simulink model "Engine_Testrig"  (R2013b)
settings: Solver=ode15s  StartTime=0.0  StopTime=100  RelTol=1e-5  AbsTol=1e-4
undefined symbols (not defined in the file): HEV_Param
libraries: fl_lib x10, nesl_utility x5, sdl_lib x1, simulink x1
Description:
  | Copyright 2015 The MathWorks, Inc.
settings Model: Creator=smiller  LastModifiedBy=smiller
settings DataIOCC: SignalLoggingSaveFormat=ModelDataLogs
settings OptimizationCC: ExpressionDepthLimit=2147483647
settings DebuggingCC: FcnCallInpInsideContextMsg=UseLocalSettings  StateNameClashWarn=warning
settings GRTTargetCC: CombineOutputUpdateFcns=off  GRTInterface=on

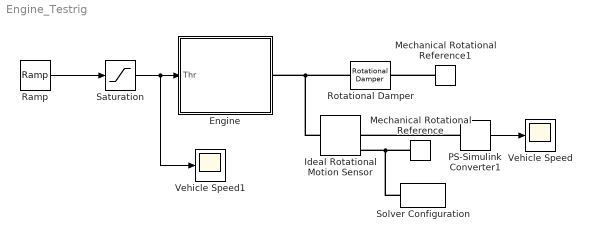
== system Engine_Testrig ==
  Engine : Subsystem
      mask Display:
      | image(imread('HEV_Engine_IMAGE.jpg'));
      | port_label('input',1,'Thr');
      | port_label('RConn',1,'Sh');
  Ideal Rotational Motion Sensor : fl_lib/Mechanical/Mechanical Sensors/Ideal Rotational Motion Sensor  offset=0 rad  w_Log=off  t_Log=off  phi_Log=off  LocalVarNames=|w|t|phi  LocalVarDescs=|w|t|phi  LocalVarLogging=[0 0 0]
  Mechanical Rotational Reference : fl_lib/Mechanical/Rotational Elements/Mechanical Rotational Reference  t_Log=off  LocalVarNames=|t  LocalVarDescs=|t  LocalVarLogging=0
  Mechanical Rotational Reference1 : fl_lib/Mechanical/Rotational Elements/Mechanical Rotational Reference  t_Log=off  LocalVarNames=|t  LocalVarDescs=|t  LocalVarLogging=0
  PS-Simulink Converter1 : nesl_utility/PS-Simulink Converter  PhysicalDomain=network_engine_domain  SubClassName=ps_output  LeftPortType=input  RightPortType=output  PseudoPeriodic=off  Frequencies=[]  Unit=rpm  AffineConversion=off
  Ramp : simulink/Sources/Ramp  slope=0.1  start=0.1  X0=0
  Rotational Damper : fl_lib/Mechanical/Rotational Elements/Rotational Damper  D=HEV_Param.ICE.Friction*0.001 N*m/(rad/s)  t_Log=off  w_Log=off  LocalVarNames=|t|w  LocalVarDescs=|t|w  LocalVarLogging=[0 0]
  Saturation : Saturate  UpperLimit=1  LowerLimit=-1
  Solver Configuration : nesl_utility/Solver Configuration  PhysicalDomain=network_engine_domain  SubClassName=solver  LeftPortType=input  RightPortType=generic  Accelerate=off  Tones=[]  Harmonics=[]  SimulateNoise=off  Profile=off  UseLocalSampling=off  EnableSwitchedLinearOptims=on  FrequencyDomain=off  UseCCode=off  RelTol=0.001  AbsTol=1e-06  MinStep=1e-09  ToWorkspace=off  DoDC=off  ResidualTolerance=1e-9  UseLocalSolver=off  LocalSolverChoice=NE_BACKWARD_EULER_ADVANCER  LocalSolverSampleTime=0.005  DoFixedCost=off  MaxNonlinIter=3  MaxModeIter=2  LinearAlgebra=Sparse  DelaysMemoryBudget=1024
  Vehicle Speed : Scope
      settings: YMin=0  YMax=120  Decimation=decimation
  Vehicle Speed1 : Scope
      settings: YMin=0  YMax=120  Decimation=decimation
  wires:
  Ramp/1 -> Saturation/1
  Saturation/1 -> Engine/1(Thr), Vehicle Speed1/1
  PS-Simulink Converter1/1 -> Vehicle Speed/1
  connections:
  Ideal Rotational Motion Sensor/LConn1 -- Engine/RConn1 -- Rotational Damper/LConn1
  Mechanical Rotational Reference1/LConn1 -- Rotational Damper/RConn1
  PS-Simulink Converter1/LConn1 -- Ideal Rotational Motion Sensor/RConn2
  Mechanical Rotational Reference/LConn1 -- Ideal Rotational Motion Sensor/RConn1 -- Solver Configuration/RConn1

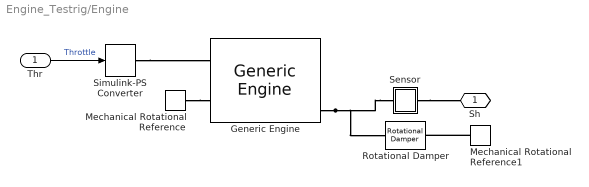
== system Engine_Testrig/Engine ==
  Thr : Inport
  Generic Engine : sdl_lib/Engines/Generic Engine  model_parameterization=1  engine_type=1  P_max=HEV_Param.ICE.Max_Power W  w_P_max=HEV_Param.ICE.Speed_At_Max_Power rpm  w_max=HEV_Param.ICE.Max_Speed rpm  w_min=500 rpm  w_tab=[ 500 1000 2e+3 3e+3 4e+3 5e+3 6e+3 7e+3 ] rpm  trq_tab=[ 380 380 380 380 350 280 200 80 ] N*m  pwr_tab=[ 2e+4 4e+4 7.8e+4 1.2e+5 1.45e+5 1.48e+5 1.25e+5 6e+4 ] W  interp_method=1  model_inertia=1  inertia=HEV_Param.ICE.Shaft_Inertia kg*m^2  initial_velocity=800 rpm  model_time_constant=0  time_constant=0.2 s  T0=0  w_thr=100 rpm  idle_speed=0  idle_speed_reference=1000 rpm  tau_controller=1 s  idle_w_thr=1 rpm  fc_model=1  fc_per_rev=25 mg/rev  displaced_volume=400 cm^3  rev_per_cycle=2  fc_w_tab=[ 1000 2e+3 3e+3 4e+3 5e+3 6e+3 ] rpm  fc_trq_tab=[ 0 80 160 200 240 320 360 400 ] N*m  fc_tab=[ 0.5 0.9 1.4 1.6 1.9 2.7 3.4 4.4; 1 1.7 2.7 3.1 3.6 5 6 7.4; 1.4 2.7 4 4.8 5.6 7.5 8.5 10.5; 2 3.6 5.8 6.7 8 10.4 11.7 13.3; 2.5 4.8 7.9 9.4 10.8 14 16.2 18.6; 3.1 6 10.3 11.9 13.8 18.4 22 26.5 ] g/s  bmep_tab=[ 0 250 500 625 750 1000 1.15e+3 1.25e+3 ] kPa  bsfc_tab=[ 410 380 300 280 270 290 320 380; 410 370 290 270 260 270 285 320; 415 380 290 275 265 270 270 300; 420 390 310 290 285 280 280 285; 430 410 340 320 310 300 310 320; 450 430 370 340 330 330 350 380 ] g/hr/kW  fc_interp_method=1  LocalVarLogging=[]
  Mechanical Rotational Reference : fl_lib/Mechanical/Rotational Elements/Mechanical Rotational Reference  t_Log=off  LocalVarNames=|t  LocalVarDescs=|t  LocalVarLogging=0
  Mechanical Rotational Reference1 : fl_lib/Mechanical/Rotational Elements/Mechanical Rotational Reference  t_Log=off  LocalVarNames=|t  LocalVarDescs=|t  LocalVarLogging=0
  Rotational Damper : fl_lib/Mechanical/Rotational Elements/Rotational Damper  D=HEV_Param.ICE.Friction N*m/(rad/s)  t_Log=off  w_Log=off  LocalVarNames=|t|w  LocalVarDescs=|t|w  LocalVarLogging=[0 0]
  Sensor : Subsystem
      mask Display: disp('S');
  Simulink-PS Converter : nesl_utility/Simulink-PS Converter  PhysicalDomain=network_engine_domain  SubClassName=ps_input  LeftPortType=input  RightPortType=output  PseudoPeriodic=off  Frequencies=[]  NoiseDistribution=none  NoiseParameters=[]  Unit=1  AffineConversion=off  InputFiltering=off  SimscapeFilterOrder=1  InputFilterTimeConstant=.001  UdotUserProvided=0
  Sh : PMIOPort  Port=1  Side=Right
  wires:
  Thr/1 -> Simulink-PS Converter/1  "Throttle"
  connections:
  Simulink-PS Converter/RConn1 -- Generic Engine/LConn1
  Mechanical Rotational Reference1/LConn1 -- Rotational Damper/RConn1
  Sensor/RConn1 -- Sh/RConn1
  Mechanical Rotational Reference/LConn1 -- Generic Engine/LConn2
  Sensor/LConn1 -- Generic Engine/RConn3 -- Rotational Damper/LConn1

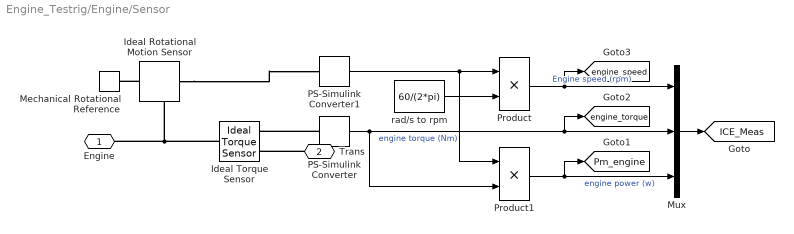
== system Engine_Testrig/Engine/Sensor ==
  Ideal Rotational Motion Sensor : fl_lib/Mechanical/Mechanical Sensors/Ideal Rotational Motion Sensor  offset=0 rad  w_Log=off  t_Log=off  phi_Log=off  LocalVarNames=|w|t|phi  LocalVarDescs=|w|t|phi  LocalVarLogging=[0 0 0]
  Ideal Torque Sensor : fl_lib/Mechanical/Mechanical Sensors/Ideal Torque Sensor  w_Log=off  t_Log=off  LocalVarNames=|w|t  LocalVarDescs=|w|t  LocalVarLogging=[0 0]
  Mechanical Rotational Reference : fl_lib/Mechanical/Rotational Elements/Mechanical Rotational Reference  t_Log=off  LocalVarNames=|t  LocalVarDescs=|t  LocalVarLogging=0
  Mux : Mux  Inputs=3
  PS-Simulink Converter : nesl_utility/PS-Simulink Converter  PhysicalDomain=network_engine_domain  SubClassName=ps_output  LeftPortType=input  RightPortType=output  PseudoPeriodic=off  Frequencies=[]  Unit=N*m  AffineConversion=off
  PS-Simulink Converter1 : nesl_utility/PS-Simulink Converter  PhysicalDomain=network_engine_domain  SubClassName=ps_output  LeftPortType=input  RightPortType=output  PseudoPeriodic=off  Frequencies=[]  Unit=rad/s  AffineConversion=off
  Product : Product  RndMeth=Zero
  Product1 : Product  RndMeth=Zero
  rad/s to rpm : Constant  Value=60/(2*pi)
  Engine : PMIOPort  Port=1  Side=Left
  Trans : PMIOPort  Port=2  Side=Right
  tag scope: ICE_Meas=global, Pm_engine=global, engine_speed=global, engine_torque=global
  wires:
  Mux/1 -> [ICE_Meas]
  rad/s to rpm/1 -> Product/2
  PS-Simulink Converter1/1 -> Product1/1, Product/1
  Product/1 -> [engine_speed], Mux/1  "Engine speed (rpm)"
  Product1/1 -> [Pm_engine], Mux/3  "engine power (w)"
  PS-Simulink Converter/1 -> [engine_torque], Mux/2, Product1/2  "engine torque (Nm)"
  connections:
  Ideal Rotational Motion Sensor/RConn2 -- PS-Simulink Converter1/LConn1
  Ideal Rotational Motion Sensor/LConn1 -- Mechanical Rotational Reference/LConn1
  PS-Simulink Converter/LConn1 -- Ideal Torque Sensor/RConn2
  Trans/RConn1 -- Ideal Torque Sensor/RConn1
  Ideal Torque Sensor/LConn1 -- Engine/RConn1 -- Ideal Rotational Motion Sensor/RConn1
